simulink model "ddv_decoupling_model"  (R2024a)
settings: Solver=VariableStepAuto  StartTime=0.0  StopTime=60  RelTol=1e-3
model workspace (MAT data in the model file):
  d = 0.5
  epsilon = 0.5
settings Model: Creator=radnor  LastModifiedBy=radnor

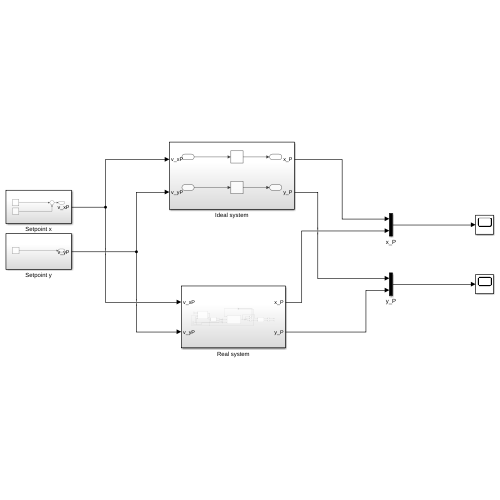
[thumbnail: Simulink's stored preview of the top-level diagram]
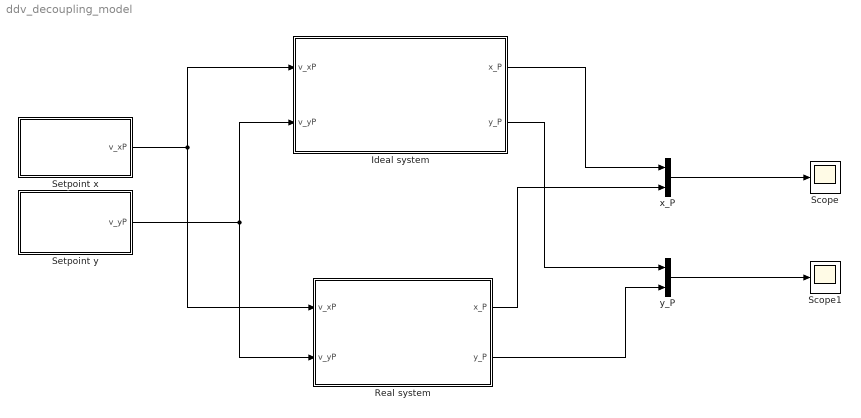
== system ddv_decoupling_model ==
  Ideal system : Subsystem
  Real system : Subsystem
  Scope : Scope
  Scope1 : Scope
  Setpoint x : Subsystem
  Setpoint y : Subsystem
  x_P : Mux  Inputs=2
  y_P : Mux  Inputs=2
  wires:
  Setpoint x/1(v_xP) -> Real system/1(v_xP), Ideal system/1(v_xP)
  Setpoint y/1(v_yP) -> Ideal system/2(v_yP), Real system/2(v_yP)
  Ideal system/1(x_P) -> x_P/1
  Real system/1(x_P) -> x_P/2
  Ideal system/2(y_P) -> y_P/1
  Real system/2(y_P) -> y_P/2
  x_P/1 -> Scope/1
  y_P/1 -> Scope1/1

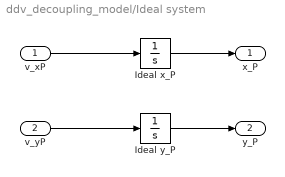
== system ddv_decoupling_model/Ideal system ==
  v_xP : Inport
  v_yP : Inport  Port=2
  Ideal x_P : Integrator
  Ideal y_P : Integrator
  x_P : Outport
  y_P : Outport  Port=2
  wires:
  Ideal y_P/1 -> y_P/1
  v_xP/1 -> Ideal x_P/1
  Ideal x_P/1 -> x_P/1
  v_yP/1 -> Ideal y_P/1

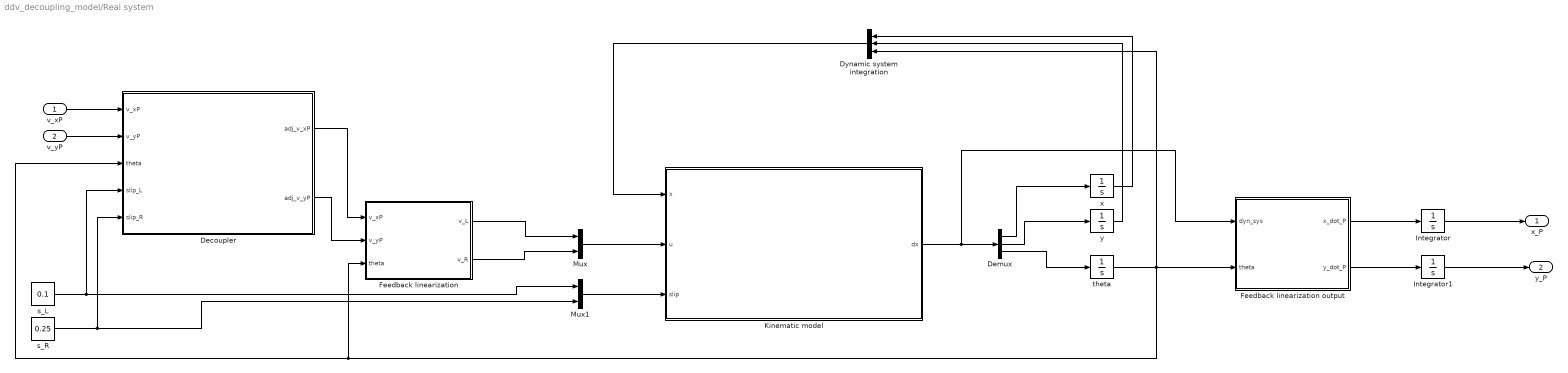
== system ddv_decoupling_model/Real system ==
  v_xP : Inport
  v_yP : Inport  Port=2
  Decoupler : MATLAB Function  TreatAsAtomicUnit=on
  Demux : Demux  Outputs=3
  Dynamic system integration : Mux  Inputs=3
  Feedback linearization : MATLAB Function  TreatAsAtomicUnit=on
  Feedback linearization output : MATLAB Function  TreatAsAtomicUnit=on
  Integrator : Integrator
  Integrator1 : Integrator
  Kinematic model : MATLAB Function  TreatAsAtomicUnit=on
  Mux : Mux  Inputs=2
  Mux1 : Mux  Inputs=2
  s_L : Constant  Value=0.1
  s_R : Constant  Value=0.25
  theta : Integrator
  x : Integrator
  y : Integrator
  x_P : Outport
  y_P : Outport  Port=2
  wires:
  Integrator1/1 -> y_P/1
  Integrator/1 -> x_P/1
  Feedback linearization output/1(x_dot_P) -> Integrator/1
  Feedback linearization output/2(y_dot_P) -> Integrator1/1
  Kinematic model/1(dx) -> Feedback linearization output/1(dyn_sys), Demux/1
  Demux/1 -> x/1
  Demux/2 -> y/1
  Demux/3 -> theta/1
  theta/1 -> Dynamic system integration/3, Feedback linearization/3(theta), Decoupler/3(theta), Feedback linearization output/2(theta)
  Mux/1 -> Kinematic model/2(u)
  Feedback linearization/1(v_L) -> Mux/1
  Feedback linearization/2(v_R) -> Mux/2
  Mux1/1 -> Kinematic model/3(slip)
  s_L/1 -> Decoupler/4(slip_L), Mux1/1
  s_R/1 -> Decoupler/5(slip_R), Mux1/2
  x/1 -> Dynamic system integration/1
  y/1 -> Dynamic system integration/2
  Dynamic system integration/1 -> Kinematic model/1(x)
  Decoupler/2(adj_v_yP) -> Feedback linearization/2(v_yP)
  Decoupler/1(adj_v_xP) -> Feedback linearization/1(v_xP)
  v_xP/1 -> Decoupler/1(v_xP)
  v_yP/1 -> Decoupler/2(v_yP)

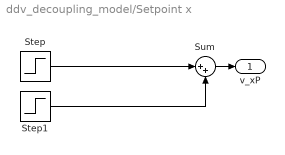
== system ddv_decoupling_model/Setpoint x ==
  Step : Step  Time=5  SampleTime=0
  Step1 : Step  Time=10  SampleTime=0
  Sum : Sum  Inputs=|++
  v_xP : Outport
  wires:
  Step/1 -> Sum/1
  Step1/1 -> Sum/2
  Sum/1 -> v_xP/1

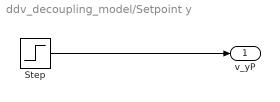
== system ddv_decoupling_model/Setpoint y ==
  Step : Step  Time=30  SampleTime=0
  v_yP : Outport
  wires:
  Step/1 -> v_yP/1

== matlab function ddv_decoupling_model/Real system/Feedback linearization output ==
  data: dyn_sys input; x_dot_P output; theta input; y_dot_P output; epsilon parameter
function [x_dot_P, y_dot_P] = fl_output(dyn_sys, theta, epsilon)
    x_dot = dyn_sys(1);
    y_dot = dyn_sys(2);
    theta_dot = dyn_sys(3);

    x_dot_P = x_dot - epsilon*theta_dot*sin(theta);
    y_dot_P = y_dot + epsilon*theta_dot*cos(theta);
end

== matlab function ddv_decoupling_model/Real system/Kinematic model ==
  data: x input; u input; dx output size=3; slip input; d parameter
function dx = kinematic_model(x, u, slip, d)
    v_L = u(1);
    v_R = u(2);
    theta = x(3);

    eta_L = 1-slip(1);
    eta_R = 1-slip(2);

    dx = zeros(3,1);
    dx(1) = 0.5*eta_R*cos(theta)*v_R + 0.5*eta_L*cos(theta)*v_L;
    dx(2) = 0.5*eta_R*sin(theta)*v_R + 0.5*eta_L*sin(theta)*v_L;
    dx(3) = 0.5*eta_R*v_R/d - 0.5*eta_L*v_L/d;
end

== matlab function ddv_decoupling_model/Real system/Feedback linearization ==
  data: v_xP input; v_L output; v_yP input; v_R output; theta input; d parameter; epsilon parameter
function [v_L, v_R] = ddv_feedback_linearization(v_xP, v_yP, theta, d, epsilon)

    v_x = v_xP*cos(theta) + v_yP*sin(theta);
    omega = 1/epsilon*(-v_xP*sin(theta) + v_yP*cos(theta));

    v_L = v_x - d*omega;
    v_R = v_x + d*omega;

end

== matlab function ddv_decoupling_model/Real system/Decoupler ==
  data: v_xP input; adj_v_xP output; v_yP input; theta input; slip_L input; slip_R input; adj_v_yP output
function [adj_v_xP, adj_v_yP] = decouple(v_xP, v_yP, theta, slip_L, slip_R)
    eta_L = 1-slip_L;
    eta_R = 1-slip_R;

    d11 = eta_R/2*(1+sin(2*theta))+eta_L/2*(1-sin(2*theta));
    d12 = -(eta_R-eta_L)/2*cos(2*theta);
    d21 = d12;
    d22 = eta_R/2*(1-sin(2*theta))+eta_L/2*(1+sin(2*theta));

    adj_v_xP = 1/(eta_R*eta_L)*(d11*v_xP+d12*v_yP);
    adj_v_yP = 1/(eta_R*eta_L)*(d21*v_xP+d22*v_yP);
end
